simulink model "airplane_EPS"  (Simulink 7.6)
settings: Solver=ode45  StartTime=0.0  StopTime=10  RelTol=1e-3
undefined symbols (not defined in the file or in its folder): DiscIntNeverNeededParam
settings Model: Creator=Jiwei  LastModifiedBy=Administrator
settings OptimizationCC: ExpressionDepthLimit=128
settings CodeAppCC: CustomSymbolStrType=$N$R$M_T
settings GRTTargetCC: CombineOutputUpdateFcns=on

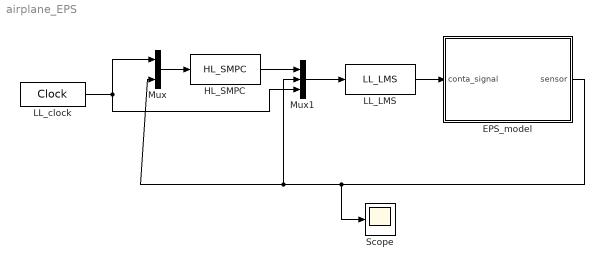
== system airplane_EPS ==
  EPS_model : Subsystem
  HL_SMPC : MATLABFcn  MATLABFcn=HL_SMPC  OutputDimensions=27
  LL_LMS : MATLABFcn  MATLABFcn=LL_LMS  OutputDimensions=26
  LL_clock : DigitalClock
  Mux : Mux  Inputs=2
  Mux1 : Mux  Inputs=3
  Scope : Scope
  wires:
  LL_clock/1 -> Mux1/3, Mux/1
  Mux/1 -> HL_SMPC/1
  HL_SMPC/1 -> Mux1/1
  LL_LMS/1 -> EPS_model/1(conta_signal)
  Mux1/1 -> LL_LMS/1
  EPS_model/1(sensor) -> Scope/1, Mux/2, Mux1/2

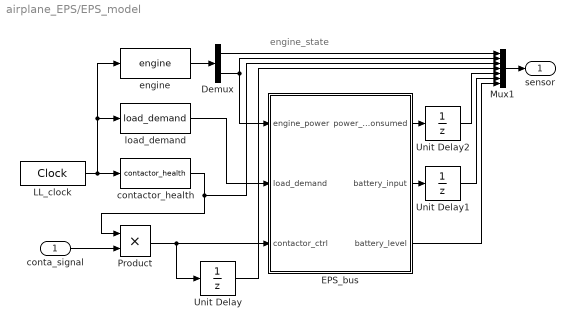
== system airplane_EPS/EPS_model ==
  note: engine_state
  conta_signal : Inport
  Demux : Demux  Outputs=[3 3]
  EPS_bus : Subsystem
  LL_clock : DigitalClock
  Mux1 : Mux  Inputs=7
  Product : Product
  Unit Delay : UnitDelay  SampleTime=-1
  Unit Delay1 : UnitDelay  SampleTime=-1
  Unit Delay2 : UnitDelay  SampleTime=-1
  contactor_health : MATLABFcn  MATLABFcn=contactor_health  OutputDimensions=26
  engine : MATLABFcn  MATLABFcn=engine  OutputDimensions=6
  load_demand : MATLABFcn  MATLABFcn=load_demand  OutputDimensions=40
  sensor : Outport
  wires:
  engine/1 -> Demux/1
  load_demand/1 -> EPS_bus/2(load_demand)
  LL_clock/1 -> contactor_health/1, engine/1, load_demand/1
  conta_signal/1 -> Product/2
  Product/1 -> EPS_bus/3(contactor_ctrl), Unit Delay/1
  Demux/1 -> Mux1/1
  Demux/2 -> Mux1/2, EPS_bus/1(engine_power)
  contactor_health/1 -> Mux1/3, Product/1
  EPS_bus/3(battery_level) -> Mux1/7
  Mux1/1 -> sensor/1
  Unit Delay/1 -> Mux1/4
  EPS_bus/1(power_consumed) -> Unit Delay2/1
  EPS_bus/2(battery_input) -> Unit Delay1/1
  Unit Delay1/1 -> Mux1/6
  Unit Delay2/1 -> Mux1/5

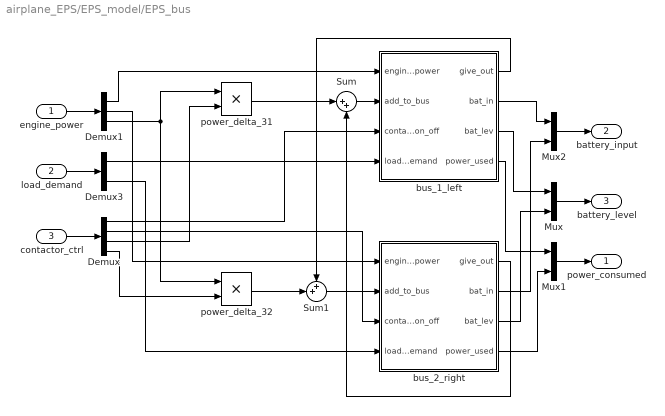
== system airplane_EPS/EPS_model/EPS_bus ==
  engine_power : Inport
  load_demand : Inport  Port=2
  contactor_ctrl : Inport  Port=3
  Demux : Demux  Outputs=[12 12 1 1]
  Demux1 : Demux  Outputs=[1 1 1]
  Demux3 : Demux  Outputs=[20 20]
  Mux : Mux  Inputs=2
  Mux1 : Mux  Inputs=2
  Mux2 : Mux  Inputs=2
  Sum : Sum  Inputs=|++
  Sum1 : Sum  Inputs=++|
  bus_1_left : Subsystem
  bus_2_right : Subsystem
  power_delta_31 : Product
  power_delta_32 : Product
  power_consumed : Outport
  battery_input : Outport  Port=2
  battery_level : Outport  Port=3
  wires:
  contactor_ctrl/1 -> Demux/1
  engine_power/1 -> Demux1/1
  Demux1/1 -> bus_1_left/1(engine_power)
  Demux1/2 -> bus_2_right/1(engine_power)
  Demux/1 -> bus_1_left/3(contactor_on_off)
  Demux/2 -> bus_2_right/3(contactor_on_off)
  load_demand/1 -> Demux3/1
  Demux3/2 -> bus_2_right/4(load_demand)
  Demux3/1 -> bus_1_left/4(load_demand)
  Mux/1 -> battery_level/1
  bus_1_left/3(bat_lev) -> Mux/1
  bus_2_right/3(bat_lev) -> Mux/2
  Sum/1 -> bus_1_left/2(add_to_bus)
  bus_2_right/1(give_out) -> Sum/2
  Sum1/1 -> bus_2_right/2(add_to_bus)
  bus_1_left/1(give_out) -> Sum1/1
  power_delta_31/1 -> Sum/1
  power_delta_32/1 -> Sum1/2
  Demux/3 -> power_delta_31/2
  Demux/4 -> power_delta_32/2
  Demux1/3 -> power_delta_32/1, power_delta_31/1
  Mux1/1 -> power_consumed/1
  bus_1_left/4(power_used) -> Mux1/1
  bus_2_right/4(power_used) -> Mux1/2
  Mux2/1 -> battery_input/1
  bus_1_left/2(bat_in) -> Mux2/1
  bus_2_right/2(bat_in) -> Mux2/2

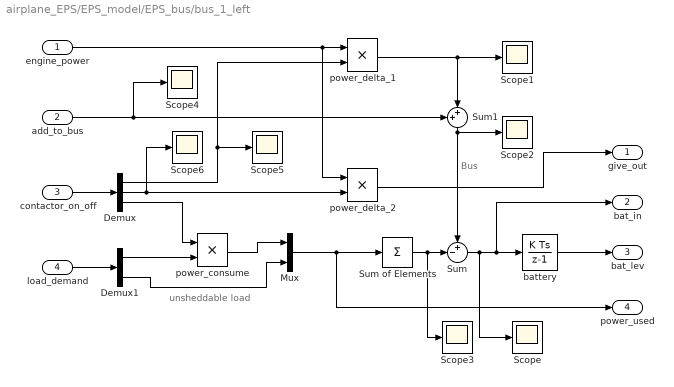
== system airplane_EPS/EPS_model/EPS_bus/bus_1_left ==
  note: unsheddable load
  note: Bus
  engine_power : Inport
  add_to_bus : Inport  Port=2
  contactor_on_off : Inport  Port=3
  load_demand : Inport  Port=4
  Demux : Demux  Outputs=[1 1 10]
  Demux1 : Demux  Outputs=[10 10]
  Mux : Mux  Inputs=2
  Scope{,1..6} (7 alike) : Scope
      Scope1 settings: SaveName=ScopeData2
      Scope2 settings: SaveName=ScopeData3
      Scope3 settings: SaveName=ScopeData4
      Scope4 settings: SaveName=ScopeData9
      Scope5 settings: SaveName=ScopeData10
      Scope6 settings: SaveName=ScopeData11
  Sum : Sum  Inputs=+-|
  Sum of Elements : Sum  Inputs=+
  Sum1 : Sum  Inputs=++|
  battery : DiscreteIntegrator  InitialCondition=45  LimitOutput=on  UpperSaturationLimit=200  LowerSaturationLimit=0  ICPrevOutput=DiscIntNeverNeededParam  ICPrevScaledInput=DiscIntNeverNeededParam
  power_consume : Product
  power_delta_1 : Product
  power_delta_2 : Product
  give_out : Outport
  bat_in : Outport  Port=2
  bat_lev : Outport  Port=3
  power_used : Outport  Port=4
  wires:
  power_delta_1/1 -> Sum1/2, Scope1/1
  contactor_on_off/1 -> Demux/1
  engine_power/1 -> power_delta_2/1, power_delta_1/1
  add_to_bus/1 -> Scope4/1, Sum1/1
  power_delta_2/1 -> give_out/1
  Sum1/1 -> Scope2/1, Sum/1
  Sum/1 -> Scope/1, bat_in/1, battery/1
  Sum of Elements/1 -> Scope3/1, Sum/2
  Demux/1 -> Scope5/1, power_delta_1/2
  Demux/2 -> Scope6/1, power_delta_2/2
  Demux/3 -> power_consume/1
  battery/1 -> bat_lev/1
  load_demand/1 -> Demux1/1
  Demux1/1 -> power_consume/2
  power_consume/1 -> Mux/1
  Demux1/2 -> Mux/2
  Mux/1 -> power_used/1, Sum of Elements/1

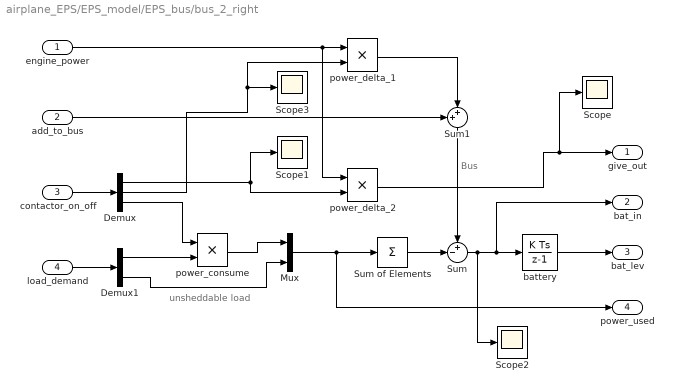
== system airplane_EPS/EPS_model/EPS_bus/bus_2_right ==
  note: unsheddable load
  note: Bus
  engine_power : Inport
  add_to_bus : Inport  Port=2
  contactor_on_off : Inport  Port=3
  load_demand : Inport  Port=4
  Demux : Demux  Outputs=[1 1 10]
  Demux1 : Demux  Outputs=[10 10]
  Mux : Mux  Inputs=2
  Scope{,1..3} (4 alike) : Scope
      Scope settings: SaveName=ScopeData5
      Scope1 settings: SaveName=ScopeData6
      Scope2 settings: SaveName=ScopeData7
      Scope3 settings: SaveName=ScopeData8
  Sum : Sum  Inputs=+-|
  Sum of Elements : Sum  Inputs=+
  Sum1 : Sum  Inputs=++|
  battery : DiscreteIntegrator  InitialCondition=45  LimitOutput=on  UpperSaturationLimit=200  LowerSaturationLimit=0  ICPrevOutput=DiscIntNeverNeededParam  ICPrevScaledInput=DiscIntNeverNeededParam
  power_consume : Product
  power_delta_1 : Product
  power_delta_2 : Product
  give_out : Outport
  bat_in : Outport  Port=2
  bat_lev : Outport  Port=3
  power_used : Outport  Port=4
  wires:
  power_delta_1/1 -> Sum1/2
  contactor_on_off/1 -> Demux/1
  engine_power/1 -> power_delta_2/1, power_delta_1/1
  add_to_bus/1 -> Sum1/1
  power_delta_2/1 -> Scope/1, give_out/1
  Sum1/1 -> Sum/1
  Sum/1 -> Scope2/1, bat_in/1, battery/1
  Sum of Elements/1 -> Sum/2
  Demux/2 -> power_delta_1/2, Scope3/1
  Demux/1 -> power_delta_2/2, Scope1/1
  Demux/3 -> power_consume/1
  battery/1 -> bat_lev/1
  load_demand/1 -> Demux1/1
  Demux1/1 -> power_consume/2
  power_consume/1 -> Mux/1
  Demux1/2 -> Mux/2
  Mux/1 -> power_used/1, Sum of Elements/1
